simulink model "manual_verification"  (R2025a)
settings: Solver=VariableStepAuto  StartTime=0.0  StopTime=1.0  RelTol=1e-3
libraries: simulink x3, mcbeeMathTransformLib x2
settings Model: Creator=brandon  LastModifiedBy=brandon

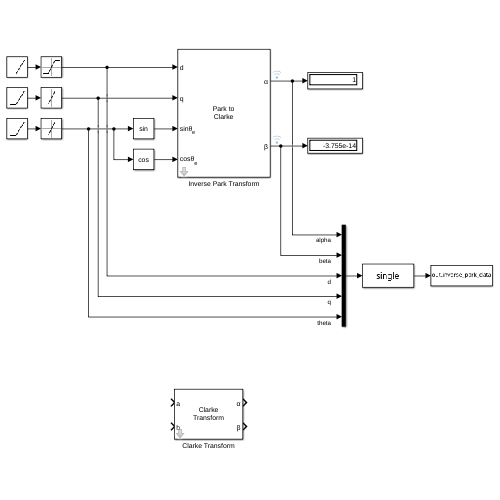
[thumbnail: Simulink's stored preview of the top-level diagram]
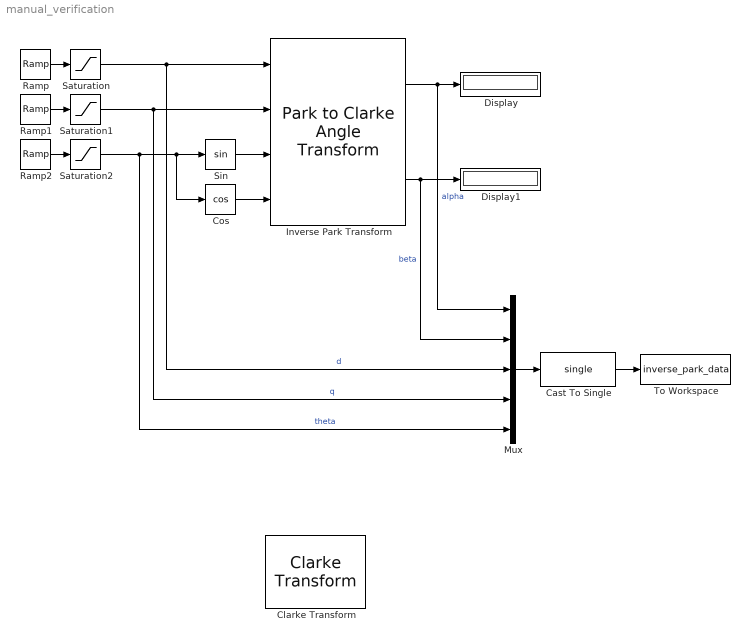
== system manual_verification ==
  Cast To Single : DataTypeConversion  OutDataTypeStr=single  SaturateOnIntegerOverflow=off  RndMeth=Floor
  Clarke Transform : mcbeeMathTransformLib/Clarke Transform  VariantControl=Variant2  PowerInvariant=off  UseWithEmbedded=on  PhaseInput=Two inputs
      settings: LibrarySourceBlock=mcbhdllib/Controls/Math Transforms/Clarke Transform
  Cos : Trigonometry  Operator=cos
  Display : Display
      settings: Decimation=6
  Display1 : Display
      settings: Decimation=6
  Inverse Park Transform : mcbeeMathTransformLib/Park to Clarke Angle Transform  AxisAlignment=D-axis  UseWithEmbedded=on  PhaseInput=Two inputs  ThetaInput=Sine and Cosine electrical position  AngleInput=Per-unit  N_points=1024
      settings: LibrarySourceBlock=mcblib/Controls/Math Transforms/Inverse Park Transform
  Mux : Mux  Inputs=5
  Ramp : simulink/Sources/Ramp  slope=1  start=0  InitialOutput=0
  Ramp1 : simulink/Sources/Ramp  slope=-1  start=0  InitialOutput=1
  Ramp2 : simulink/Sources/Ramp  slope=2*pi  start=0  InitialOutput=0
  Saturation : Saturate  UpperLimit=1.0  LowerLimit=0.0
  Saturation1 : Saturate  UpperLimit=1.0  LowerLimit=0.0
  Saturation2 : Saturate  UpperLimit=2*pi  LowerLimit=0.0
  Sin : Trigonometry
  To Workspace : ToWorkspace  VariableName=inverse_park_data  SaveFormat=Timeseries  SampleTime=-1
  wires:
  Saturation/1 -> Mux/3, Inverse Park Transform/1  "d"
  Inverse Park Transform/1 -> Mux/1, Display/1  "alpha"
  Inverse Park Transform/2 -> Mux/2, Display1/1  "beta"
  Saturation1/1 -> Mux/4, Inverse Park Transform/2  "q"
  Cos/1 -> Inverse Park Transform/4
  Sin/1 -> Inverse Park Transform/3
  Saturation2/1 -> Mux/5, Cos/1, Sin/1  "theta"
  Mux/1 -> Cast To Single/1
  Cast To Single/1 -> To Workspace/1
  Ramp/1 -> Saturation/1
  Ramp1/1 -> Saturation1/1
  Ramp2/1 -> Saturation2/1
